simulink model "ATRover"  (R2017b)
settings: configuration reference "Config_IC_Sil" (kept outside this file)
settings Model: RequirementInfo={} %GIDa_ade1690c_d179_406e_b5c5_07040df803cc  DataDictionary=RoverDataDict.sldd  Creator=zwqe6u  LastModifiedBy=eh6qym
settings ConfigSetRef: DDName=RoverDataDict.sldd

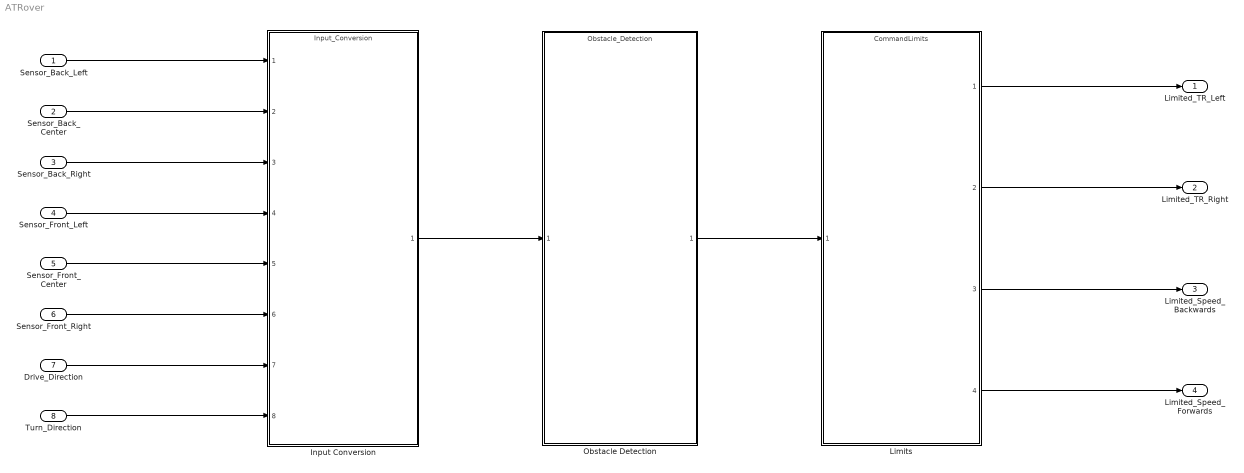
== system ATRover ==
  Sensor_Back_Left : Inport  OutDataTypeStr=double  PortDimensions=1
  Sensor_Back_Center : Inport  Port=2  OutDataTypeStr=double  PortDimensions=1
  Sensor_Back_Right : Inport  Port=3  OutDataTypeStr=double  PortDimensions=1
  Sensor_Front_Left : Inport  Port=4  OutDataTypeStr=double  PortDimensions=1
  Sensor_Front_Center : Inport  Port=5  OutDataTypeStr=double  PortDimensions=1
  Sensor_Front_Right : Inport  Port=6  OutDataTypeStr=double  PortDimensions=1
  "Drive_Direction " : Inport  Port=7  OutDataTypeStr=double
  Turn_Direction : Inport  Port=8  OutDataTypeStr=double
  Input Conversion : ModelReference  RequirementInfo={} %GIDa_929bd00e_6027_4e27_b4a1_78e6b9f55a0d  ModelNameDialog=Input_Conversion.slx  SimulationMode=Normal  ModelReferenceVersion=1.136
  Limits : ModelReference  RequirementInfo={} %GIDa_b8795b12_60fc_4210_a280_232d13fa426e  ModelNameDialog=CommandLimits.slx  SimulationMode=Normal  ModelReferenceVersion=1.133
  Obstacle Detection : ModelReference  RequirementInfo={} %GIDa_96683e72_6301_411e_abda_9ddf50a246a2  ModelNameDialog=Obstacle_Detection.slx  SimulationMode=Normal  ModelReferenceVersion=1.149
  Limited_TR_Left : Outport  OutDataTypeStr=double
  Limited_TR_Right : Outport  Port=2  OutDataTypeStr=double
  Limited_Speed_Backwards : Outport  Port=3  OutDataTypeStr=double
  Limited_Speed_Forwards : Outport  Port=4  OutDataTypeStr=double
  wires:
  Sensor_Back_Left/1 -> Input Conversion/1
  Sensor_Back_Center/1 -> Input Conversion/2
  Sensor_Back_Right/1 -> Input Conversion/3
  Sensor_Front_Left/1 -> Input Conversion/4
  Sensor_Front_Center/1 -> Input Conversion/5
  Sensor_Front_Right/1 -> Input Conversion/6
  "Drive_Direction "/1 -> Input Conversion/7
  Turn_Direction/1 -> Input Conversion/8
  Obstacle Detection/1 -> Limits/1
  Limits/1 -> Limited_TR_Left/1
  Limits/2 -> Limited_TR_Right/1
  Limits/3 -> Limited_Speed_Backwards/1
  Limits/4 -> Limited_Speed_Forwards/1
  Input Conversion/1 -> Obstacle Detection/1
